simulink model "S_fcn_trig_step"  (R2020a)
settings: Solver=FixedStepDiscrete  StartTime=0.0  StopTime=10.0  FixedStep=5e-6  RelTol=1e-3
settings Model: Creator=anony  LastModifiedBy=anony

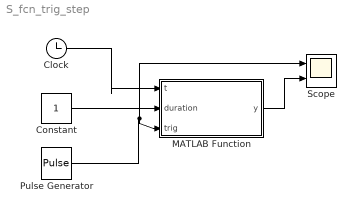
== system S_fcn_trig_step ==
  Clock : Clock
  Constant : Constant
  MATLAB Function : MATLAB Function  TreatAsAtomicUnit=on
  Pulse Generator : DiscretePulseGenerator  PulseType=Time based  Period=1.2
  Scope : Scope  NumInputPorts=2
  wires:
  Clock/1 -> MATLAB Function/1(t)
  Pulse Generator/1 -> Scope/1, MATLAB Function/3(trig)
  MATLAB Function/1(y) -> Scope/2
  Constant/1 -> MATLAB Function/2(duration)

== matlab function S_fcn_trig_step/MATLAB Function ==
  data: t input; duration input; y output; trig input
function y = fcn(t, duration, trig)

persistent trig_now trig_last t_start state_change
    if isempty(trig_now)
        trig_now = 0;
    end

    if isempty(trig_last)
        trig_last = 0;
    end
    
    if isempty(t_start)
        t_start = 0;
    end
    
    
    if isempty(state_change)
        state_change = 0;
    end

trig_now = trig;
if trig_now ~= trig_last
    state_change = 1;
    t_start = t;
end

if state_change == 1
    if t - t_start > duration
        state_change = 0;
    end
end

trig_last = trig_now;
y = state_change;
